simulink model "Rotor_hub"  (R2015a)
settings: Solver=ode45  StartTime=0.0  StopTime=10.0  RelTol=1e-3
undefined symbols (not defined in the file or in its folder): b, i, I_Pi, K_q, K_t
libraries: aerolibutil x2
settings Model: Creator=Mattia  LastModifiedBy=Claudio

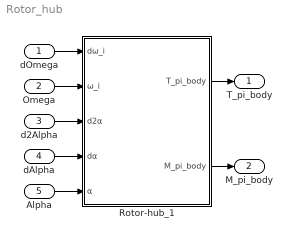
== system Rotor_hub ==
  dOmega : Inport
  Omega : Inport  Port=2
  d2Alpha : Inport  Port=3
  dAlpha : Inport  Port=4
  Alpha : Inport  Port=5
  Rotor-hub_1 : Subsystem
  " T_pi_body" : Outport
  " M_pi_body" : Outport  Port=2
  wires:
  Omega/1 -> Rotor-hub_1/2(ω_i)
  dOmega/1 -> Rotor-hub_1/1(dω_i)
  Alpha/1 -> Rotor-hub_1/5(α)
  dAlpha/1 -> Rotor-hub_1/4(dα)
  d2Alpha/1 -> Rotor-hub_1/3(d2α)
  Rotor-hub_1/1(" T_pi_body") -> " T_pi_body"/1
  Rotor-hub_1/2(" M_pi_body") -> " M_pi_body"/1

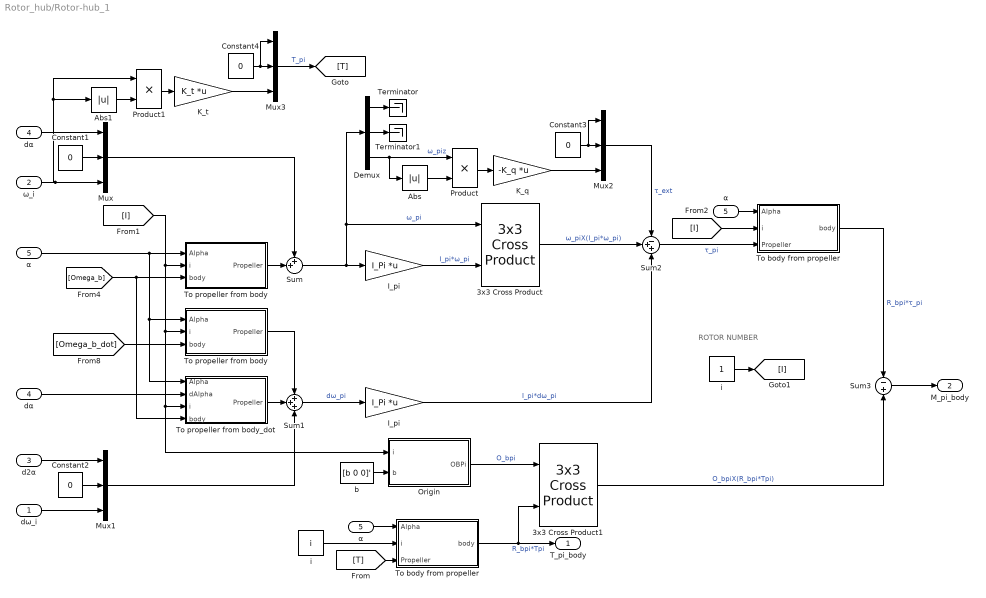
== system Rotor_hub/Rotor-hub_1 ==
  note: ROTOR NUMBER
  dω_i : Inport
  ω_i : Inport  Port=2
  d2α : Inport  Port=3
  dα : Inport  Port=4
  α : Inport  Port=5
  3x3 Cross Product : aerolibutil/3x3 Cross Product
  3x3 Cross Product1 : aerolibutil/3x3 Cross Product
  Abs : Abs
  Abs1 : Abs
  Constant{1..4} (4 alike) : Constant  Value=0
  Demux : Demux  Outputs=3
  I_pi : Gain  Gain=I_Pi  Multiplication=Matrix(K*u)
  "I_pi " : Gain  Gain=I_Pi  Multiplication=Matrix(K*u)
  K_q : Gain  Gain=-K_q  Multiplication=Matrix(K*u)
  K_t : Gain  Gain=K_t  Multiplication=Matrix(K*u)
  Mux{,1..3} (4 alike) : Mux  Inputs=3
  Origin : MATLAB Function  TreatAsAtomicUnit=on
  Product : Product
  Product1 : Product
  Sum : Sum  Inputs=++|
  Sum1 : Sum  Inputs=+++
  Sum2 : Sum  Inputs=-++
  Sum3 : Sum  Inputs=-|+
  Terminator : Terminator
  Terminator1 : Terminator
  To body from propeller : MATLAB Function  TreatAsAtomicUnit=on
  "To body from propeller " : MATLAB Function  TreatAsAtomicUnit=on
  To propeller from body : MATLAB Function  TreatAsAtomicUnit=on
  "To propeller from body " : MATLAB Function  TreatAsAtomicUnit=on
  To propeller from body_dot : MATLAB Function  TreatAsAtomicUnit=on
  b : Constant  Value=[b 0 0]'
  "dα " : InportShadow  Port=4
  i : Constant
  "i " : Constant  Value=i
  "α " : InportShadow  Port=5
  "α  " : InportShadow  Port=5
  " T_pi_body" : Outport
  " M_pi_body" : Outport  Port=2
  wires:
  α/1 -> To propeller from body/1(Alpha), "To propeller from body "/1(Alpha), To propeller from body_dot/1(Alpha)
  [Omega_b] -> To propeller from body/3(body), To propeller from body_dot/4(body)
  [I] -> Origin/1(i), To propeller from body_dot/3(i), "To propeller from body "/2(i), To propeller from body/2(i)
  Constant1/1 -> Mux/2
  Sum/1 -> Demux/1, 3x3 Cross Product/1, "I_pi "/1  "ω_pi"
  Constant2/1 -> Mux1/2
  [Omega_b_dot] -> "To propeller from body "/3(body)
  To propeller from body_dot/1(Propeller) -> Sum1/2
  Sum1/1 -> I_pi/1  "dω_pi"
  Mux1/1 -> Sum1/3
  To propeller from body/1(Propeller) -> Sum/2
  Mux/1 -> Sum/1
  "To propeller from body "/1(Propeller) -> Sum1/1
  "I_pi "/1 -> 3x3 Cross Product/2  "I_pi*ω_pi"
  3x3 Cross Product/1 -> Sum2/2  "ω_piX(I_pi*ω_pi)"
  I_pi/1 -> Sum2/3  "I_pi*dω_pi"
  Mux2/1 -> Sum2/1  "τ_ext"
  Constant3/1 -> Mux2/1, Mux2/2
  K_q/1 -> Mux2/3
  Demux/1 -> Terminator/1
  Demux/2 -> Terminator1/1
  Demux/3 -> Abs/1, Product/1  "ω_piz"
  Product/1 -> K_q/1
  Abs/1 -> Product/2
  Product1/1 -> K_t/1
  Abs1/1 -> Product1/2
  b/1 -> Origin/2(b)
  "α "/1 -> To body from propeller/1(Alpha)
  "i "/1 -> To body from propeller/2(i)
  "dα "/1 -> To propeller from body_dot/2(dAlpha)
  Origin/1(OBPi) -> 3x3 Cross Product1/1  "O_bpi"
  [T] -> To body from propeller/3(Propeller)
  To body from propeller/1(body) -> 3x3 Cross Product1/2, " T_pi_body"/1  "R_bpi*Tpi"
  3x3 Cross Product1/1 -> Sum3/2  "O_bpiX(R_bpi*Tpi)"
  "α  "/1 -> "To body from propeller "/1(Alpha)
  [I] -> "To body from propeller "/2(i)
  Sum2/1 -> "To body from propeller "/3(Propeller)  "τ_pi"
  "To body from propeller "/1(body) -> Sum3/1  "R_bpi*τ_pi"
  Sum3/1 -> " M_pi_body"/1
  i/1 -> [I]
  dα/1 -> Mux/1
  ω_i/1 -> Product1/1, Abs1/1, Mux/3
  Constant4/1 -> Mux3/1, Mux3/2
  Mux3/1 -> [T]  "T_pi"
  K_t/1 -> Mux3/3
  d2α/1 -> Mux1/1
  dω_i/1 -> Mux1/3

== matlab function Rotor_hub/Rotor-hub_1/To propeller from body  ==
  data: Alpha input; i input; Propeller output; body input
 function Propeller = RPiB(Alpha, i, body)
%#codegen
Salpha = sin(Alpha);
Calpha = cos(Alpha);

psi = (1-i)*pi/2;
Spsi = sin(psi);
Cpsi = cos(psi);

Rx = [1     0      0   ; 
      0  Calpha Salpha ; 
      0 -Salpha Calpha]; 
Rz = [ Cpsi Spsi 0 ;
      -Spsi Cpsi 0 ; 
        0    0   1];
    
RBPi = Rz*Rx;
RPiB = RBPi';

Propeller = RPiB * body;

== matlab function Rotor_hub/Rotor-hub_1/To propeller from body ==
  data: Alpha input; i input; Propeller output; body input
 function Propeller = RPiB(Alpha, i, body)
%#codegen
Salpha = sin(Alpha);
Calpha = cos(Alpha);

psi = (1-i)*pi/2;
Spsi = sin(psi);
Cpsi = cos(psi);

Rx = [1     0      0   ; 
      0  Calpha Salpha ; 
      0 -Salpha Calpha]; 
Rz = [ Cpsi Spsi 0 ;
      -Spsi Cpsi 0 ; 
        0    0   1];
    
RBPi = Rz*Rx;
RPiB = RBPi';

Propeller = RPiB * body;

== matlab function Rotor_hub/Rotor-hub_1/To propeller from body_dot ==
  data: Alpha input; dAlpha input; i input; Propeller output; body input
 function Propeller = RPiB_dot(Alpha,dAlpha, i, body)
%#codegen
Salpha = sin(Alpha);
Calpha = cos(Alpha);

psi = (1-i)*pi/2;
Spsi = sin(psi);
Cpsi = cos(psi);

Rx = [1     0      0   ; 
      0  Calpha Salpha ; 
      0 -Salpha Calpha]; 
Rxdot = dAlpha*[0     0       0   ; 
                0 -Salpha  Calpha ; 
                0 -Calpha -Salpha];  
  
Rz = [ Cpsi Spsi 0 ;
      -Spsi Cpsi 0 ; 
        0    0   1];
    
RBPidot = Rz*Rxdot;
RPiBdot = RBPidot'

Propeller = RPiBdot* body;

== matlab function Rotor_hub/Rotor-hub_1/Origin ==
  data: i input; b input; OBPi output
function OBPi = R_zi(i, b)
%#codegen
psi = (1-i)*pi/2;
Spsi = sin(psi);
Cpsi = cos(psi);

Rz = [ Cpsi Spsi 0 ;
      -Spsi Cpsi 0 ; 
        0    0   1];
    
RBPi = Rz;

OBPi = RBPi * b;

== matlab function Rotor_hub/Rotor-hub_1/To body from propeller ==
  data: Alpha input; i input; Propeller input; body output
 function body = RBPi(Alpha, i, Propeller)
%#codegen
Salpha = sin(Alpha);
Calpha = cos(Alpha);

psi = (1-i)*pi/2;
Spsi = sin(psi);
Cpsi = cos(psi);

Rx = [1     0      0   ; 
      0  Calpha Salpha ; 
      0 -Salpha Calpha]; 
Rz = [ Cpsi Spsi 0 ;
      -Spsi Cpsi 0 ; 
        0    0   1];
    
RBPi = Rz*Rx;

body = RBPi * Propeller;

== matlab function Rotor_hub/Rotor-hub_1/To body from propeller  ==
  data: Alpha input; i input; Propeller input; body output
 function body = RBPi(Alpha, i, Propeller)
%#codegen
Salpha = sin(Alpha);
Calpha = cos(Alpha);

psi = (1-i)*pi/2;
Spsi = sin(psi);
Cpsi = cos(psi);

Rx = [1     0      0   ; 
      0  Calpha Salpha ; 
      0 -Salpha Calpha]; 
Rz = [ Cpsi Spsi 0 ;
      -Spsi Cpsi 0 ; 
        0    0   1];
    
RBPi = Rz*Rx;

body = RBPi * Propeller;
